simulink model "JoshTestingOCTModel"  (R2018b)
settings: Solver=VariableStepAuto  StartTime=0.0  StopTime=simParams.duration.Value  FixedStep=0.01  MaxStep=0.1*sqrt(simParams.lengthScaleFactor.Value)  RelTol=1e-3  AbsTol=1e-3
undefined symbols (not defined in the file): dragTurbine, dragTurbine_ul, env, flightController, FLIGHTCONTROLLER, flightController_cl, fltCtrl, fluidDynamicSurface, fluidDynamicSurface_cl, fuselage, fuselage_cl, initializeBussesFromBlock, initializeVariantsFromBlock, pathFollowingController, pathFollowingController_cl, plant, plant_cl, sixDoFDynamics, sixDoFDynamics_cl, sixDoFDynamicsCoupled, surfaceCoefficients, surfaceCoefficients_ul, tethersMoment, tethersMoment_cl, thrAttachPtKinematics, thrAttachPtKinematics_ul, vehicle, vehicle_cl, vehicleLE, vehicleLE_cl, vhcl
libraries: vrlib x18, dspstat3 x3, vectorNormalizer_ul x3, localApparentWind_ul x3, xProdMatrix_ul x2, dynamicPressure_ul x2, dsppolyfun x2, animation_cl x1, environment_cl x1, oneTetherThreeSurfaceCtrl_cl x1, courseFollow_cl x1, ctrlAllocMatrixLE_cl x1
(part 1 of 2)
PreSaveFcn:
  | % Callback to reset the view so that the
  | % the next person to open isn't totally lost.
  | hilite_system('OCTModel/plant');
  | hilite_system('OCTModel/plant','none');
  | set_param(gcs,'Zoomfactor','fit to view')
settings Model: SimulationMode=accelerator  ExtModeTrigDuration=100  Creator=mcobb  LastModifiedBy=jldanie5
settings SolverCC: AlgebraicLoopSolver=LineSearch  SolverResetMethod=Robust
settings DataIOCC: SaveOutput=off  DSMLogging=off  StateSaveName=tmp_raccel_xout
settings OptimizationCC: EfficientMapNaN2IntZero=off
settings DebuggingCC: SignalRangeChecking=error  AlgebraicLoopMsg=none  ArtificialAlgebraicLoopMsg=none
settings HardwareCC: TargetBitPerPointer=64  TargetBitPerSizeT=64  TargetBitPerPtrDiffT=64  TargetLongLongMode=on  TargetIntDivRoundTo=Zero  TargetEndianess=LittleEndian  TargetWordSize=64  TargetHWDeviceType=MATLAB Host  ProdEqTarget=off
settings CodeAppCC: MaxIdLength=128
settings GRTTargetCC: TargetLangStandard=C89/C90 (ANSI)  CombineOutputUpdateFcns=off  GRTInterface=on

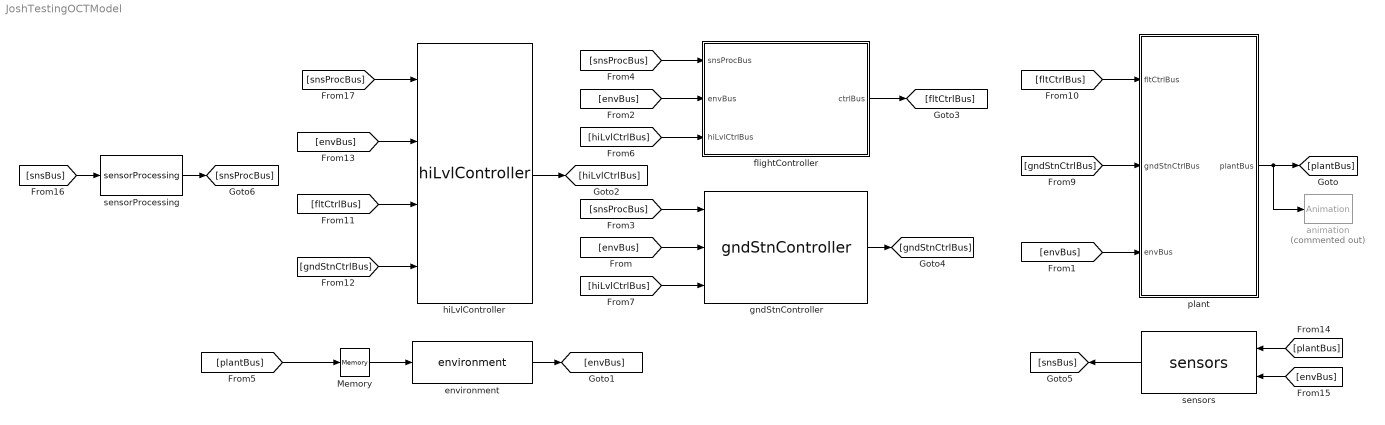
== system JoshTestingOCTModel ==
  Memory : Memory
  animation : animation_cl/Animation  Commented=on  animSampleTime=0.1  scaleFactor=scaleFactor  elevation=45  radius=500  vidLogEnbl=off  vidDims=[240 480]*2
  environment : environment_cl/environment  SystemSampleTime=-1
  flightController : Subsystem  AncestorBlock=flightController_cl/flightController  LoadFcn=initializeVariantsFromBlock(gcb)  InitFcn=initializeVariantsFromBlock(gcb)  StartFcn=initializeVariantsFromBlock(gcb)  Variant=on
      settings: PreSaveFcn=initializeVariantsFromBlock(gcb)
  gndStnController : gndStnController_cl/gndStnController  SystemSampleTime=-1
      link override anchorTetherCtrl: ctrl=gndCtrl
  hiLvlController : hiLvlController_cl/hiLvlController  SystemSampleTime=-1
  plant : Subsystem  AncestorBlock=plant_cl/plant  LoadFcn=initializeBussesFromBlock(gcb)  InitFcn=initializeBussesFromBlock(gcb)  StartFcn=initializeBussesFromBlock(gcb)  VariantControl=VSS_plant_modularPlant
  sensorProcessing : sensorProcessing_cl/sensorProcessing  SystemSampleTime=-1
  sensors : sensors_cl/sensors  SystemSampleTime=-1
  wires:
  environment/1 -> [envBus]
  [envBus] -> gndStnController/2
  [envBus] -> plant/3(envBus)
  [snsProcBus] -> gndStnController/1
  [snsProcBus] -> flightController/1(snsProcBus)
  [snsProcBus] -> hiLvlController/1
  flightController/1(ctrlBus) -> [fltCtrlBus]
  gndStnController/1 -> [gndStnCtrlBus]
  [gndStnCtrlBus] -> plant/2(gndStnCtrlBus)
  [fltCtrlBus] -> plant/1(fltCtrlBus)
  [envBus] -> hiLvlController/2
  [fltCtrlBus] -> hiLvlController/3
  [gndStnCtrlBus] -> hiLvlController/4
  [plantBus] -> Memory/1
  [hiLvlCtrlBus] -> flightController/3(hiLvlCtrlBus)
  [hiLvlCtrlBus] -> gndStnController/3
  plant/1(plantBus) -> [plantBus], animation/1
  hiLvlController/1 -> [hiLvlCtrlBus]
  Memory/1 -> environment/1
  [envBus] -> flightController/2(envBus)
  [plantBus] -> sensors/1
  [envBus] -> sensors/2
  sensors/1 -> [snsBus]
  [snsBus] -> sensorProcessing/1
  sensorProcessing/1 -> [snsProcBus]

== system JoshTestingOCTModel/flightController ==
  snsProcBus : Inport  OutDataTypeStr=Bus: sensorsProcessingBus
  envBus : Inport  Port=2  OutDataTypeStr=Bus: envBus
  hiLvlCtrlBus : Inport  Port=3  OutDataTypeStr=Bus: hiLvlCtrlBus
  oneTetherThreeSurfaceCtrl : oneTetherThreeSurfaceCtrl_cl/oneTetherThreeSurfaceCtrl  SystemSampleTime=-1  VariantControl=strcmpi(FLIGHTCONTROLLER,'oneTetherThreeSurfaceCtrl')
  pathFollowingController : Subsystem  AncestorBlock=pathFollowingController_cl/pathFollowingController  LoadFcn=initializeBussesFromBlock(gcb)  InitFcn=initializeBussesFromBlock(gcb)  StartFcn=initializeBussesFromBlock(gcb)  VariantControl=strcmpi(FLIGHTCONTROLLER,'pathFollowingController')  mask{initPosForInitSStar=vhcl.initPosVecGnd.Value, fluidDensity=env.water.density.Value, pathCtrl=fltCtrl, aeroStruct=vhcl.struct('OCT.aeroSurfLE')}
      mask prompts: initPosForInitSStar "Initial Position"; fluidDensity "Fluid Density"; pathCtrl "Controller"; aeroStruct "Aerodynamic Structure"
      settings: MinAlgLoopOccurrences=on
      mask DialogControl Container3 Prompt: courseFollow Params
      mask DialogControl Container4 Prompt: setpointToOutput Params
  takeoffToLanding : takeoffToLanding_cl/takeoffToLanding  VariantControl=strcmpi(FLIGHTCONTROLLER,'takeoffToLanding')  initPosForInitSStar=vhcl.initPosVecGnd.Value  fluidDensity=env.water.density.Value  pathCtrl=fltCtrl  aeroStruct=vhcl.struct('OCT.aeroSurf')
  threeTetherThreeSurfaceCtrl : threeTetherThreeSurfaceCtrl_cl/threeTetherThreeSurfaceCtrl  VariantControl=strcmpi(FLIGHTCONTROLLER,'threeTetherThreeSurfaceCtrl')  ctrl=fltCtrl
  ctrlBus : Outport  OutDataTypeStr=Bus: fltCtrlBus

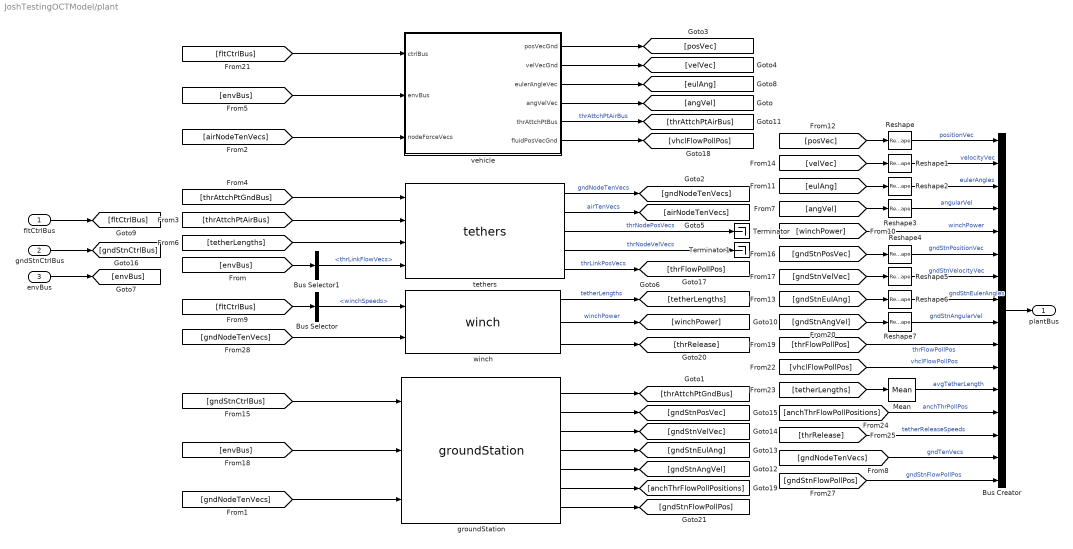
== system JoshTestingOCTModel/plant ==
  fltCtrlBus : Inport  OutDataTypeStr=Bus: fltCtrlBus
  gndStnCtrlBus : Inport  Port=2  OutDataTypeStr=Bus: gndStnCtrlBus
  envBus : Inport  Port=3  OutDataTypeStr=Bus: envBus
  Bus Creator : BusCreator  Inputs=16  OutDataTypeStr=Bus: plantBus  NonVirtualBus=on
  Bus Selector : BusSelector  OutputSignals=winchSpeeds
  Bus Selector1 : BusSelector  OutputSignals=thrLinkFlowVecs
  Mean : dspstat3/Mean  run=off  InputProcessing=Columns as channels (frame based)  reset_popup=None  directionMode=Each column  dimension=1  roiEnable=off  roiType=Rectangles  roiPortion=Entire ROI  roiOutput=Individual statistics for each ROI  roiFlag=off  roundingMode=Floor  overflowMode=off  outputDataTypeStr=Inherit: Same as accumulator  outputMin=[]  outputMax=[]  outputLastDataTypeStr=Inherit: Same as accumulator
  Reshape{,1..7} (8 alike) : Reshape  OutputDimensionality=Column vector (2-D)
  Terminator : Terminator
  Terminator1 : Terminator
  groundStation : groundStation_cl/groundStation  numNodes=2
  tethers : tethers_cl/tethers  SystemSampleTime=-1
  vehicle : Subsystem  AncestorBlock=vehicle_cl/vehicle  LoadFcn=initializeVariantsFromBlock(gcb)  InitFcn=initializeVariantsFromBlock(gcb)  StartFcn=initializeVariantsFromBlock(gcb)  Variant=on
      settings: PreSaveFcn=initializeVariantsFromBlock(gcb)
  winch : winch_cl/winch  SystemSampleTime=-1
  plantBus : Outport  OutDataTypeStr=Bus: plantBus
  wires:
  [gndNodeTenVecs] -> winch/2
  tethers/5 -> [thrFlowPollPos]  "thrLinkPosVecs"
  [gndStnFlowPollPos] -> Bus Creator/16  "gndStnFlowPollPos"
  groundStation/7 -> [gndStnFlowPollPos]
  [gndNodeTenVecs] -> Bus Creator/15  "gndTenVecs"
  [thrRelease] -> Bus Creator/14  "tetherReleaseSpeeds"
  [anchThrFlowPollPositions] -> Bus Creator/13  "anchThrPollPos"
  groundStation/6 -> [anchThrFlowPollPositions]
  Mean/1 -> Bus Creator/12  "avgTetherLength"
  [tetherLengths] -> Mean/1
  Bus Selector1/1 -> tethers/4  "<thrLinkFlowVecs>"
  [vhclFlowPollPos] -> Bus Creator/11  "vhclFlowPollPos"
  vehicle/6(fluidPosVecGnd) -> [vhclFlowPollPos]
  [thrFlowPollPos] -> Bus Creator/10  "thrFlowPollPos"
  tethers/4 -> Terminator1/1  "thrNodeVelVecs"
  winch/3 -> [thrRelease]
  Bus Selector/1 -> winch/1  "<winchSpeeds>"
  gndStnCtrlBus/1 -> [gndStnCtrlBus]
  groundStation/5 -> [gndStnAngVel]
  groundStation/4 -> [gndStnEulAng]
  groundStation/3 -> [gndStnVelVec]
  groundStation/2 -> [gndStnPosVec]
  Reshape7/1 -> Bus Creator/9  "gndStnAngularVel"
  Reshape6/1 -> Bus Creator/8  "gndStnEulerAngles"
  Reshape5/1 -> Bus Creator/7  "gndStnVelocityVec"
  Reshape4/1 -> Bus Creator/6  "gndStnPositionVec"
  [gndStnPosVec] -> Reshape4/1
  [gndStnVelVec] -> Reshape5/1
  [gndStnEulAng] -> Reshape6/1
  [gndStnAngVel] -> Reshape7/1
  [winchPower] -> Bus Creator/5  "winchPower"
  winch/2 -> [winchPower]  "winchPower"
  Reshape3/1 -> Bus Creator/4  "angularVel"
  [angVel] -> Reshape3/1
  [fltCtrlBus] -> Bus Selector/1
  [envBus] -> vehicle/2(envBus)
  [fltCtrlBus] -> vehicle/1(ctrlBus)
  [gndStnCtrlBus] -> groundStation/1
  [envBus] -> groundStation/2
  [tetherLengths] -> tethers/3
  [thrAttchPtGndBus] -> tethers/1
  [thrAttchPtAirBus] -> tethers/2
  [airNodeTenVecs] -> vehicle/3(nodeForceVecs)
  [gndNodeTenVecs] -> groundStation/3
  tethers/3 -> Terminator/1  "thrNodePosVecs"
  tethers/2 -> [airNodeTenVecs]  "airTenVecs"
  tethers/1 -> [gndNodeTenVecs]  "gndNodeTenVecs"
  groundStation/1 -> [thrAttchPtGndBus]
  [envBus] -> Bus Selector1/1
  vehicle/4(angVelVec) -> [angVel]
  vehicle/2(velVecGnd) -> [velVec]
  vehicle/5(thrAttchPtBus) -> [thrAttchPtAirBus]  "thrAttchPtAirBus"
  vehicle/1(posVecGnd) -> [posVec]
  vehicle/3(eulerAngleVec) -> [eulAng]
  [eulAng] -> Reshape2/1
  [velVec] -> Reshape1/1
  [posVec] -> Reshape/1
  winch/1 -> [tetherLengths]  "tetherLengths"
  Reshape1/1 -> Bus Creator/2  "velocityVec"
  Reshape2/1 -> Bus Creator/3  "eulerAngles"
  Reshape/1 -> Bus Creator/1  "positionVec"
  Bus Creator/1 -> plantBus/1
  fltCtrlBus/1 -> [fltCtrlBus]
  envBus/1 -> [envBus]

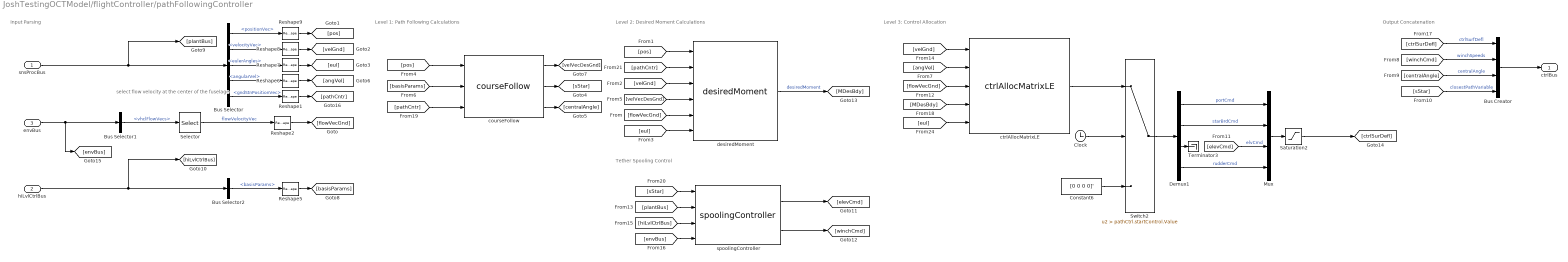
== system JoshTestingOCTModel/flightController/pathFollowingController ==
  note: Input Parsing
  note: Level 1: Path Following Calculations
  note: Level 2: Desired Moment Calculations
  note: Tether Spooling Control
  note: Output Concatenation
  note: Level 3: Control Allocation
  note: select flow velocity at the center of the fuselage
  snsProcBus : Inport  OutDataTypeStr=Bus: sensorsProcessingBus
  hiLvlCtrlBus : Inport  Port=2  OutDataTypeStr=Bus: hiLvlCtrlBus
  envBus : Inport  Port=3  OutDataTypeStr=Bus: envBus
  Bus Creator : BusCreator  Inputs=4  OutDataTypeStr=Bus: fltCtrlBus
      settings: InheritFromInputs=off
  Bus Selector : BusSelector  OutputSignals=positionVec,velocityVec,eulerAngles,angularVel,gndStnPositionVec
  Bus Selector1 : BusSelector  OutputSignals=vhclFlowVecs
  Bus Selector2 : BusSelector  OutputSignals=basisParams
  Clock : Clock
  Constant6 : Constant  Value=[0 0 0 0]'
  Demux1 : Demux
  Mux : Mux
  Reshape{1..2,5..9} (7 alike) : Reshape  OutputDimensionality=Column vector (2-D)
  Saturation2 : Saturate  UpperLimit=pathCtrl.controlSigMax.upperLimit.Value  LowerLimit=pathCtrl.controlSigMax.lowerLimit.Value
  Selector : Selector  NumberOfDimensions=2  InputPortWidth=3  IndexOptions=Select all,Index vector (dialog)  Indices=[1 3],5  OutputSizes=1,1
  Switch2 : Switch  Criteria=u2 > Threshold  Threshold=pathCtrl.startControl.Value
  Terminator3 : Terminator
  courseFollow : courseFollow_cl/courseFollow  SystemSampleTime=-1
  ctrlAllocMatrixLE : ctrlAllocMatrixLE_cl/ctrlAllocMatrixLE  aeroStruct=aeroStruct  fluidDensity=fluidDensity  ctrlUpMax=pathCtrl.controlSigMax.upperLimit.Value  ctrlDnMax=pathCtrl.controlSigMax.lowerLimit.Value
  desiredMoment : setpointToOutput_cl/desiredMoment  SystemSampleTime=-1
  spoolingController : spoolingController_cl/spoolingController  SystemSampleTime=-1
  ctrlBus : Outport  OutDataTypeStr=Bus: fltCtrlBus
  wires:
  [basisParams] -> courseFollow/2
  [flowVecGnd] -> desiredMoment/5
  [eul] -> desiredMoment/6
  [velVecDesGnd] -> desiredMoment/4
  [velGnd] -> desiredMoment/3
  [pathCntr] -> desiredMoment/2
  [pos] -> desiredMoment/1
  [pathCntr] -> courseFollow/3
  Bus Selector/5 -> Reshape1/1  "<gndStnPositionVec>"
  Reshape1/1 -> [pathCntr]
  [envBus] -> spoolingController/4
  spoolingController/2 -> [winchCmd]
  spoolingController/1 -> [elevCmd]
  Bus Selector1/1 -> Selector/1  "<vhclFlowVecs>"
  [hiLvlCtrlBus] -> spoolingController/3
  [plantBus] -> spoolingController/2
  [sStar] -> spoolingController/1
  envBus/1 -> Bus Selector1/1, [envBus]
  Selector/1 -> Reshape2/1  "flowVelocityVec"
  [eul] -> ctrlAllocMatrixLE/5
  Reshape9/1 -> [pos]
  Reshape8/1 -> [velGnd]
  Reshape7/1 -> [eul]
  Reshape6/1 -> [angVel]
  Reshape2/1 -> [flowVecGnd]
  Saturation2/1 -> [ctrlSurDefl]
  Reshape5/1 -> [basisParams]
  Bus Selector2/1 -> Reshape5/1  "<basisParams>"
  [ctrlSurDefl] -> Bus Creator/1  "ctrlSurfDefl"
  ctrlAllocMatrixLE/1 -> Switch2/1
  [MDesBdy] -> ctrlAllocMatrixLE/4
  Constant6/1 -> Switch2/3
  Switch2/1 -> Demux1/1
  Clock/1 -> Switch2/2
  Demux1/2 -> Mux/2  "starBrdCmd"
  Demux1/1 -> Mux/1  "portCmd"
  Demux1/4 -> Mux/4  "rudderCmd"
  Demux1/3 -> Terminator3/1
  Mux/1 -> Saturation2/1
  [elevCmd] -> Mux/3  "elvCmd"
  [flowVecGnd] -> ctrlAllocMatrixLE/3
  [velGnd] -> ctrlAllocMatrixLE/1
  [angVel] -> ctrlAllocMatrixLE/2
  Bus Selector/4 -> Reshape6/1  "<angularVel>"
  desiredMoment/1 -> [MDesBdy]  "desiredMoment"
  courseFollow/3 -> [centralAngle]
  [sStar] -> Bus Creator/4  "closestPathVariable"
  [centralAngle] -> Bus Creator/3  "centralAngle"
  hiLvlCtrlBus/1 -> Bus Selector2/1, [hiLvlCtrlBus]
  courseFollow/2 -> [sStar]
  [winchCmd] -> Bus Creator/2  "winchSpeeds"
  Bus Creator/1 -> ctrlBus/1
  [pos] -> courseFollow/1
  Bus Selector/3 -> Reshape7/1  "<eulerAngles>"
  Bus Selector/1 -> Reshape9/1  "<positionVec>"
  Bus Selector/2 -> Reshape8/1  "<velocityVec>"
  snsProcBus/1 -> Bus Selector/1, [plantBus]
  courseFollow/1 -> [velVecDesGnd]

== system JoshTestingOCTModel/plant/vehicle ==
  ctrlBus : Inport  OutDataTypeStr=Bus: fltCtrlBus
  envBus : Inport  Port=2  OutDataTypeStr=Bus: envBus
  nodeForceVecs : Inport  Port=3
  vehicle000 : vehicle000_cl/vehicle000  VariantControl=VSS_vehicle_vehicle000  vcl=vhcl  rho=env.water.density.Value  grav=env.gravAccel.Value
  vehicleLETest : Subsystem  AncestorBlock=vehicleLE_cl/vehicleLE  VariantControl=VSS_vehicle_vehicleLETest  mask{vcl=vhcl, rho=env.water.density.Value, grav=env.gravAccel.Value}
      mask prompts: vcl "Vehicle"; rho "Density"; grav "Gravity"
      mask DialogControl Container9 Prompt: General
      mask DialogControl Container5 Prompt: Vehicle object (OCT.vehicle)
      mask DialogControl ParameterGroupVar Prompt: Environment Object (OCT.env)
      mask Display:
      | image('kite.jpg',[100 100 601 528]/4,'on')
      | 
      | port_label('input',1,'ctrlBus')
      | port_label('input',2,'envBus')
      | port_label('input',3,'nodeForceVecs')
      | 
      | port_label('output',1,'posVecGnd')
      | port_label('output',2,'velVecGnd')
      | port_label('output',3,'eulAng')
      | port_label('output',4,'angVelVec')
      | port_label('output',5,'thrAttchPtBus')
      | port_label('output',6,'fluidPosVecGnd')
  posVecGnd : Outport
  velVecGnd : Outport  Port=2
  eulerAngleVec : Outport  Port=3
  angVelVec : Outport  Port=4
  thrAttchPtBus : Outport  Port=5
  fluidPosVecGnd : Outport  Port=6

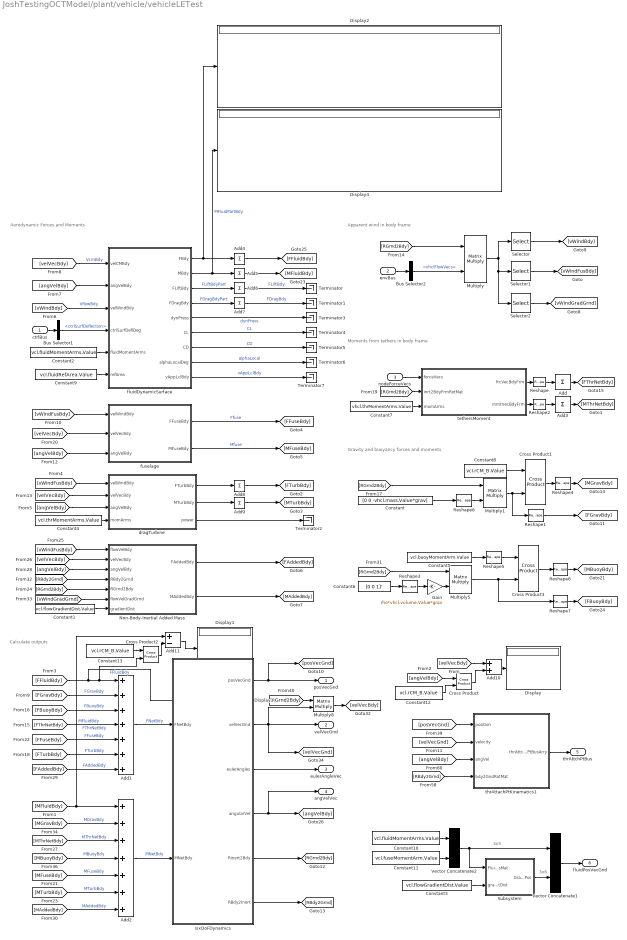
== system JoshTestingOCTModel/plant/vehicle/vehicleLETest ==
  note: Aerodynamic Forces and Moments
  note: Moments from tethers in body frame
  note: Gravity and buoyancy forces and moments
  note: Apparent wind in body frame
  note: Calculate outputs
  note: 3x5
  note: 3x6
  ctrlBus : Inport  OutDataTypeStr=Bus: fltCtrlBus
  envBus : Inport  Port=2  OutDataTypeStr=Bus: envBus
  nodeForceVecs : Inport  Port=3
  Add : Sum  Inputs=+  CollapseMode=Specified dimension  CollapseDim=2
  Add1 : Sum  Inputs=+++++++
  Add10 : Sum
  Add11 : Sum  Inputs=+-
  Add2 : Sum  Inputs=+++++++
  Add3 : Sum  Inputs=+  CollapseMode=Specified dimension  CollapseDim=2
  Add{4..9} (6 alike) : Sum  Inputs=1  CollapseMode=Specified dimension  CollapseDim=2
  Bus Selector1 : BusSelector  OutputSignals=ctrlSurfDeflection
  Bus Selector2 : BusSelector  OutputSignals=vhclFlowVecs
  Constant : Constant  Value=[0 0 -vhcl.mass.Value*grav]
  Constant1 : Constant  Value=vcl.flowGradientDist.Value
  Constant10 : Constant  Value=vcl.fluidMomentArms.Value
  Constant11 : Constant  Value=vcl.fuseMomentArm.Value
  Constant12 : Constant  Value=vcl.rCM_B.Value
  Constant13 : Constant  Value=vcl.rCM_B.Value
  Constant2 : Constant  Value=vcl.fluidMomentArms.Value
  Constant3 : Constant  Value=vcl.flowGradientDist.Value
  Constant4 : Constant  Value=vcl.thrMomentArms.Value  VectorParams1D=off
  Constant5 : Constant  Value=vcl.buoyMomentArm.Value
  Constant6 : Constant  Value=[0 0 1]'
  Constant7 : Constant  Value=vhcl.thrMomentArms.Value
  Constant8 : Constant  Value=vcl.rCM_B.Value
  Constant9 : Constant  Value=vcl.fluidRefArea.Value
  Cross Product{,1..3} (4 alike) : vrlib/Utilities/Cross Product
      settings: SourceProductBaseCode=VR
  Display{,1..4} (5 alike) : Display
  Gain : Gain  Gain=rho*vhcl.volume.Value*grav
  Multiply{,1,5,8} (4 alike) : Product  Multiplication=Matrix(*)
  Non-Body-Inertial Added Mass : Subsystem  AncestorBlock=addedMass_cl/Non-Body-Inertial Added Mass  mask{MaMat=vcl.Ma6x6_B.Value}
      mask prompts: MaMat "Added Mass Matrix"
  Reshape : Reshape  OutputDimensionality=Customize  OutputDimensions=[3 vcl.numTethers.Value]
  Reshape{1,3..8} (7 alike) : Reshape  OutputDimensionality=Column vector (2-D)
  Reshape2 : Reshape  OutputDimensionality=Customize  OutputDimensions=[3 vcl.numTethers.Value]
  Selector : Selector  NumberOfDimensions=2  InputPortWidth=3  IndexOptions=Select all,Index vector (dialog)  Indices=[1 3],1:4  OutputSizes=1,1
  Selector1 : Selector  NumberOfDimensions=2  InputPortWidth=3  IndexOptions=Select all,Index vector (dialog)  Indices=[1 3],5  OutputSizes=1,1
  Selector2 : Selector  NumberOfDimensions=2  InputPortWidth=3  IndexOptions=Select all,Index vector (dialog)  Indices=[1 3],6:11  OutputSizes=1,1
  Subsystem : Subsystem
  Terminator{,1..7} (8 alike) : Terminator
  Vector Concatenate1 : Concatenate  Mode=Multidimensional array  ConcatenateDimension=2
  Vector Concatenate2 : Concatenate  Mode=Multidimensional array  ConcatenateDimension=2
  dragTurbine : Subsystem  AncestorBlock=dragTurbine_ul/dragTurbine  TreatAsAtomicUnit=on  mask{rho_fluid=rho, turb_struct=vcl.struct('OCT.turb'), momArms=0}
      mask prompts: rho_fluid "Fluid density"; turb_struct "Turbines structure"; momArms "Turbine Moment Arms"
  fluidDynamicSurface : Subsystem  AncestorBlock=fluidDynamicSurface_cl/fluidDynamicSurface  mask{aeroStruct=vcl.struct('OCT.aeroSurfLE'), fluidDensity=env.water.density.Value}
      mask prompts: aeroStruct "Aerodynamic surface structure"; fluidDensity "Fluid density"
      mask help:
      | Input must be an 1×N struct array with fields:
      |     refArea
      |     aeroCentPosVec
      |     spanUnitVec
      |     chordUnitVec
      |     CL
      |     CD
      |     alpha
      |     GainCL
      |     GainCD
      |
      | where N is the number of aerodynamic surfaces
      settings: MinAlgLoopOccurrences=on
  fuselage : Subsystem  AncestorBlock=fuselage_cl/fuselage  mask{momArm=vcl.fuseMomentArm.Value, fus=vcl.fuse, fusRhoDa=rho}
      mask prompts: momArm "Fuselage Moment Arm"; fus "Fuselage"; fusRhoDa "Density"
      mask DialogControl Container4 Prompt: General
      mask DialogControl Container9 Prompt: Fuselage object (OCT.fuselage)
      mask DialogControl Container8 Prompt: Environment Object (OCT.env)
  sixDoFDynamics : Subsystem  AncestorBlock=sixDoFDynamics_cl/sixDoFDynamics  LoadFcn=initializeVariantsFromBlock(gcb)  InitFcn=initializeVariantsFromBlock(gcb)  Variant=on  mask{vcl=vcl}
      mask prompts: vcl "vehicle object"
  tethersMoment : Subsystem  AncestorBlock=tethersMoment_cl/tethersMoment  mask{arms=vcl.struct('OCT.thrAttchLE')}
      mask prompts: arms "Moment arm(s)"
  thrAttachPtKinematics1 : Subsystem  AncestorBlock=thrAttachPtKinematics_ul/thrAttachPtKinematics  InitFcn=thrAttachPtKinematics_init  mask{atchPts=vcl.struct('OCT.thrAttchLE')}
      mask prompts: atchPts "Tether attachment point vec in platform frame"
      mask init:
      | thrAttachPtKinematics_init
  posVecGnd : Outport
  velVecGnd : Outport  Port=2
  eulerAngleVec : Outport  Port=3
  angVelVec : Outport  Port=4
  thrAttchPtBus : Outport  Port=5
  fluidPosVecGnd : Outport  Port=6
  wires:
  Add10/1 -> Display/1
  Cross Product/1 -> Add10/2
  [velVecBdy] -> Add10/1
  Constant12/1 -> Cross Product/2
  [angVelBdy] -> Cross Product/1
  Non-Body-Inertial Added Mass/2(MAddedBdy) -> [MAddedBdy]
  sixDoFDynamics/4(angularVel) -> angVelVec/1, [angVelBdy]
  Vector Concatenate1/1 -> fluidPosVecGnd/1
  Subsystem/1(GradientFlowPos) -> Vector Concatenate1/2
  Constant3/1 -> Subsystem/2(gradientDist)
  Vector Concatenate2/1 -> Vector Concatenate1/1, Subsystem/1(FluidCentPosMat)
  Constant11/1 -> Vector Concatenate2/2
  Constant10/1 -> Vector Concatenate2/1
  [RBdy2Grnd] -> thrAttachPtKinematics1/4(bdy2GndRotMat)
  [angVelBdy] -> thrAttachPtKinematics1/3(angVel)
  [velVecGnd] -> thrAttachPtKinematics1/2(velocity)
  [posVecGnd] -> thrAttachPtKinematics1/1(position)
  sixDoFDynamics/6(RBdy2Inert) -> [RBdy2Grnd]
  sixDoFDynamics/5(Rinert2Bdy) -> [RGrnd2Bdy]
  Add2/1 -> sixDoFDynamics/2(MNetBdy)  "MNetBdy"
  [MAddedBdy] -> Add2/7  "MAddedBdy"
  [MTurbBdy] -> Add2/6  "MTurbBdy"
  [MFuseBdy] -> Add2/5  "MFuseBdy"
  [MBuoyBdy] -> Add2/4  "MBuoyBdy"
  [MThrNetBdy] -> Add2/3  "MThrNetBdy"
  [MGravBdy] -> Add2/2  "MGravBdy"
  [MFluidBdy] -> Add11/1, Add2/1  "MFluidBdy"
  Add1/1 -> sixDoFDynamics/1(FNetBdy)  "FNetBdy"
  [FAddedBdy] -> Add1/7  "FAddedBdy"
  [FTurbBdy] -> Add1/6  "FTurbBdy"
  [FFuseBdy] -> Add1/5  "FFuseBdy"
  [FThrNetBdy] -> Add1/4  "FThrNetBdy"
  [FBuoyBdy] -> Add1/3  "FBuoyBdy"
  [FGravBdy] -> Add1/2  "FGravBdy"
  [FFluidBdy] -> Display3/1, Cross Product2/2, Add1/1  "FFluidBdy"
  Multiply8/1 -> [velVecBdy]
  [RGrnd2Bdy] -> Multiply8/1
  Selector2/1 -> [vWindGradGrnd]
  Selector1/1 -> [vWindFusBdy]
  Selector/1 -> [vWindBdy]
  Multiply/1 -> Selector1/1, Selector2/1, Selector/1
  Bus Selector2/1 -> Multiply/2  "<vhclFlowVecs>"
  envBus/1 -> Bus Selector2/1
  [RGrnd2Bdy] -> Multiply/1
  Add3/1 -> [MThrNetBdy]
  Add/1 -> [FThrNetBdy]
  Reshape2/1 -> Add3/1
  Reshape/1 -> Add/1
  tethersMoment/2(mmtVecBdyFrm) -> Reshape2/1
  tethersMoment/1(frcVecBdyFrm) -> Reshape/1
  nodeForceVecs/1 -> tethersMoment/1(forceVecs)
  [RGrnd2Bdy] -> tethersMoment/2(inrt2BdyFrmRotMat)
  Constant7/1 -> tethersMoment/3(momArms)
  Reshape4/1 -> [MGravBdy]
  Cross Product1/1 -> Reshape4/1
  Constant8/1 -> Cross Product1/1
  Reshape8/1 -> Multiply1/2
  [RGrnd2Bdy] -> Multiply1/1
  Constant/1 -> Reshape8/1
  fuselage/2(MFuseBdy) -> [MFuseBdy]  "Mfuse"
  fuselage/1(FFuseBdy) -> [FFuseBdy]  "Ffuse"
  Multiply1/1 -> Cross Product1/2, Reshape1/1
  Reshape1/1 -> [FGravBdy]
  Reshape7/1 -> [FBuoyBdy]
  Multiply5/1 -> Cross Product3/2, Reshape7/1
  Reshape6/1 -> [MBuoyBdy]
  Cross Product3/1 -> Reshape6/1
  Reshape5/1 -> Cross Product3/1
  Constant5/1 -> Reshape5/1
  Gain/1 -> Multiply5/2
  [RGrnd2Bdy] -> Multiply5/1
  Reshape3/1 -> Gain/1
  Constant6/1 -> Reshape3/1
  Non-Body-Inertial Added Mass/1(FAddedBdy) -> [FAddedBdy]
  Constant1/1 -> Non-Body-Inertial Added Mass/7(gradientDist)
  [vWindGradGrnd] -> Non-Body-Inertial Added Mass/6(flowVelGradGrnd)
  [RGrnd2Bdy] -> Non-Body-Inertial Added Mass/5(RGrnd2Bdy)
  [RBdy2Grnd] -> Non-Body-Inertial Added Mass/4(RBdy2Grnd)
  [angVelBdy] -> Non-Body-Inertial Added Mass/3(angVelBdy)
  [velVecBdy] -> Non-Body-Inertial Added Mass/2(velVecBdy)
  [vWindFusBdy] -> Non-Body-Inertial Added Mass/1("flowVelBdy ")
  dragTurbine/3(power) -> Terminator2/1
  Add9/1 -> [MTurbBdy]
  Add8/1 -> [FTurbBdy]
  dragTurbine/2(MTurbBdy) -> Add9/1
  dragTurbine/1(FTurbBdy) -> Add8/1
  Constant4/1 -> dragTurbine/4(momArms)
  [angVelBdy] -> dragTurbine/3(angVelBdy)
  [velVecBdy] -> dragTurbine/2(velVecBdy)
  [vWindFusBdy] -> dragTurbine/1(velWindBdy)
  [angVelBdy] -> fuselage/3(angVelBdy)
  [velVecBdy] -> fuselage/2(velVecBdy)
  [vWindFusBdy] -> fuselage/1(velWindBdy)
  Constant9/1 -> fluidDynamicSurface/6(refArea)
  ctrlBus/1 -> Bus Selector1/1
  Bus Selector1/1 -> fluidDynamicSurface/4(ctrlSurfDeflDeg)  "<ctrlSurfDeflection>"
  [vWindBdy] -> fluidDynamicSurface/3(velWindBdy)  "VflowBdy"
  [angVelBdy] -> fluidDynamicSurface/2(angVelBdy)
  [velVecBdy] -> fluidDynamicSurface/1(velCMBdy)  "VcmBdy"
  Add7/1 -> Terminator1/1  "FDragBdy"
  Add6/1 -> Terminator/1  "FLiftBdy"
  Add5/1 -> [MFluidBdy]
  Add4/1 -> [FFluidBdy]
  fluidDynamicSurface/9(vAppLclBdy) -> Terminator7/1  "vAppLclBdy"
  fluidDynamicSurface/8(alphaLocalDeg) -> Terminator6/1  "alphaLocal"
  fluidDynamicSurface/7(CD) -> Terminator5/1  "CD"
  fluidDynamicSurface/6(CL) -> Terminator4/1  "CL"
  fluidDynamicSurface/5(dynPress) -> Terminator3/1  "dynPress"
  fluidDynamicSurface/4(FDragBdy) -> Add7/1  "FDragBdyPart"
  fluidDynamicSurface/3(FLiftBdy) -> Add6/1  "FLiftBdyPart"
  fluidDynamicSurface/2(MBdy) -> Display4/1, Add5/1  "MFluidPartBdy"
  Constant2/1 -> fluidDynamicSurface/5(fluidMomentArms)
  fluidDynamicSurface/1(FBdy) -> Display2/1, Add4/1
  thrAttachPtKinematics1/1(thrAttchPtBusArry) -> thrAttchPtBus/1
  sixDoFDynamics/2(velVecGnd) -> velVecGnd/1, [velVecGnd], Multiply8/2
  sixDoFDynamics/1(posVecGnd) -> posVecGnd/1, [posVecGnd]
  sixDoFDynamics/3(eulerAngles) -> eulerAngleVec/1
  Cross Product2/1 -> Add11/2
  Add11/1 -> Display1/1
  Constant13/1 -> Cross Product2/1

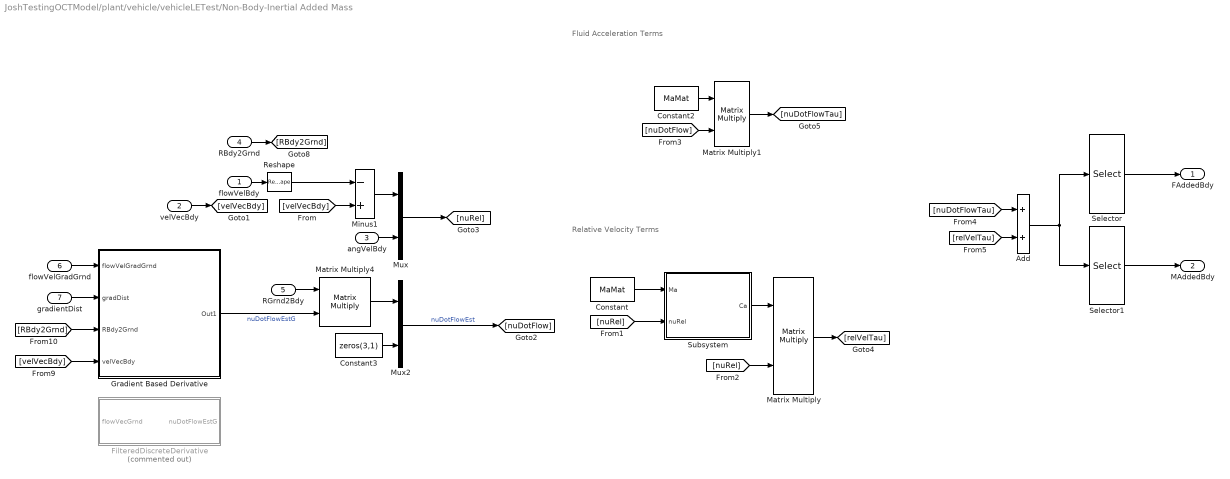
== system JoshTestingOCTModel/plant/vehicle/vehicleLETest/Non-Body-Inertial Added Mass ==
  note: Fluid Acceleration Terms
  note: Relative Velocity Terms
  "flowVelBdy " : Inport
  velVecBdy : Inport  Port=2
  angVelBdy : Inport  Port=3
  RBdy2Grnd : Inport  Port=4
  RGrnd2Bdy : Inport  Port=5
  flowVelGradGrnd : Inport  Port=6
  gradientDist : Inport  Port=7
  Add : Sum
  Constant : Constant  Value=MaMat
  Constant2 : Constant  Value=MaMat
  Constant3 : Constant  Value=zeros(3,1)
  FilteredDiscreteDerivative : Subsystem  Commented=on
  Gradient Based Derivative : Subsystem
  Matrix Multiply : Product  Multiplication=Matrix(*)
  Matrix Multiply1 : Product  Multiplication=Matrix(*)
  Matrix Multiply4 : Product  Multiplication=Matrix(*)
  Minus1 : Sum  Inputs=-+
  Mux : Mux  Inputs=2
  Mux2 : Mux  Inputs=2
  Reshape : Reshape  OutputDimensionality=Column vector (2-D)
  Selector : Selector  InputPortWidth=6  IndexOptions=Index vector (dialog)  Indices=[1 2 3]  OutputSizes=1
  Selector1 : Selector  InputPortWidth=6  IndexOptions=Index vector (dialog)  Indices=[4 5 6]  OutputSizes=1
  Subsystem : Subsystem
  FAddedBdy : Outport
  MAddedBdy : Outport  Port=2
  wires:
  Reshape/1 -> Minus1/1
  Gradient Based Derivative/1(Out1) -> Matrix Multiply4/2  "nuDotFlowEstG"
  RBdy2Grnd/1 -> [RBdy2Grnd]
  [velVecBdy] -> Gradient Based Derivative/4(velVecBdy)
  [RBdy2Grnd] -> Gradient Based Derivative/3(RBdy2Grnd)
  gradientDist/1 -> Gradient Based Derivative/2(gradDist)
  flowVelGradGrnd/1 -> Gradient Based Derivative/1(flowVelGradGrnd)
  [velVecBdy] -> Minus1/2
  velVecBdy/1 -> [velVecBdy]
  Mux/1 -> [nuRel]
  Minus1/1 -> Mux/1
  Matrix Multiply4/1 -> Mux2/1
  RGrnd2Bdy/1 -> Matrix Multiply4/1
  Mux2/1 -> [nuDotFlow]  "nuDotFlowEst"
  Constant3/1 -> Mux2/2
  Selector1/1 -> MAddedBdy/1
  Selector/1 -> FAddedBdy/1
  Add/1 -> Selector1/1, Selector/1
  [nuDotFlowTau] -> Add/1
  [relVelTau] -> Add/2
  Matrix Multiply1/1 -> [nuDotFlowTau]
  [nuDotFlow] -> Matrix Multiply1/2
  Constant2/1 -> Matrix Multiply1/1
  Matrix Multiply/1 -> [relVelTau]
  [nuRel] -> Matrix Multiply/2
  Subsystem/1(Ca) -> Matrix Multiply/1
  [nuRel] -> Subsystem/2(nuRel)
  Constant/1 -> Subsystem/1(Ma)
  "flowVelBdy "/1 -> Reshape/1
  angVelBdy/1 -> Mux/2

== system JoshTestingOCTModel/plant/vehicle/vehicleLETest/Subsystem ==
  FluidCentPosMat : Inport
  gradientDist : Inport  Port=2
  Add10 : Sum
  Constant1 : Constant  Value=ones(1,6)  VectorParams1D=off
  Constant2 : Constant  Value=eye(3)
  Gain1 : Gain  Gain=-1
  Matrix Multiply : Product  Multiplication=Matrix(*)
  Multiply2 : Product
  Selector2 : Selector  NumberOfDimensions=2  InputPortWidth=3  IndexOptions=Select all,Index vector (dialog)  Indices=[1 3],5  OutputSizes=1,1
  Vector Concatenate : Concatenate  Mode=Multidimensional array  ConcatenateDimension=2
  GradientFlowPos : Outport
  wires:
  gradientDist/1 -> Multiply2/1
  Add10/1 -> GradientFlowPos/1
  Constant2/1 -> Multiply2/2
  Gain1/1 -> Vector Concatenate/2
  Matrix Multiply/1 -> Add10/1
  Constant1/1 -> Matrix Multiply/2
  Multiply2/1 -> Vector Concatenate/1, Gain1/1
  Selector2/1 -> Matrix Multiply/1
  Vector Concatenate/1 -> Add10/2
  FluidCentPosMat/1 -> Selector2/1

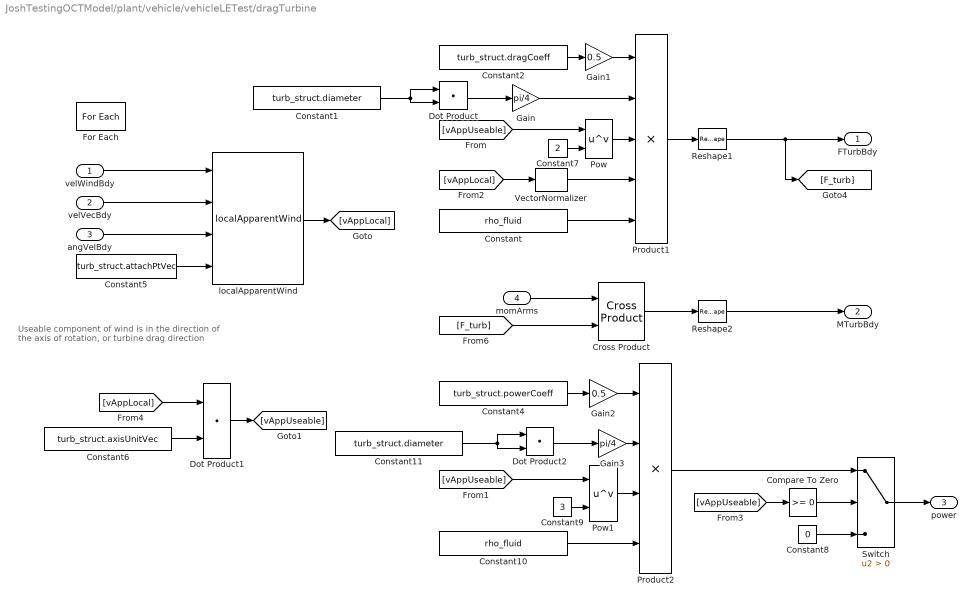
== system JoshTestingOCTModel/plant/vehicle/vehicleLETest/dragTurbine ==
  note: Useable component of wind is in the direction of
      | the axis of rotation, or turbine drag direction
  velWindBdy : Inport
  velVecBdy : Inport  Port=2
  angVelBdy : Inport  Port=3
  momArms : Inport  Port=4
  Compare To Zero : simulink/Logic and Bit Operations/Compare To Zero  relop=>=  OutDataTypeStr=boolean
  Constant : Constant  Value=rho_fluid
  Constant1 : Constant  Value=turb_struct.diameter  VectorParams1D=off
  Constant10 : Constant  Value=rho_fluid
  Constant11 : Constant  Value=turb_struct.diameter  VectorParams1D=off
  Constant2 : Constant  Value=turb_struct.dragCoeff  VectorParams1D=off
  Constant4 : Constant  Value=turb_struct.powerCoeff  VectorParams1D=off
  Constant5 : Constant  Value=turb_struct.attachPtVec
  Constant6 : Constant  Value=turb_struct.axisUnitVec
  Constant7 : Constant  Value=2
  Constant8 : Constant  Value=0
  Constant9 : Constant  Value=3
  Cross Product : vrlib/Utilities/Cross Product
      settings: SourceProductBaseCode=VR
  Dot Product : DotProduct  InputSameDT=on  OutDataTypeStr=Inherit: Inherit via internal rule
  Dot Product1 : DotProduct  InputSameDT=on  OutDataTypeStr=Inherit: Inherit via internal rule
  Dot Product2 : DotProduct  InputSameDT=on  OutDataTypeStr=Inherit: Inherit via internal rule
  For Each : ForEach  DisableCoverage=on  IterateSubsysMaskParameter=off,on,off  SubsysMaskParameterIterationDimension=1,2,1  IndexMode=One-based
  Gain : Gain  Gain=pi/4
  Gain1 : Gain  Gain=0.5
  Gain2 : Gain  Gain=0.5
  Gain3 : Gain  Gain=pi/4
  Pow : Math  Operator=pow  RndMeth=Zero  SaturateOnIntegerOverflow=on
  Pow1 : Math  Operator=pow  RndMeth=Zero  SaturateOnIntegerOverflow=on
  Product1 : Product  Inputs=5
  Product2 : Product  Inputs=4
  Reshape1 : Reshape  OutputDimensionality=Column vector (2-D)
  Reshape2 : Reshape  OutputDimensionality=Column vector (2-D)
  Switch : Switch  Criteria=u2 > Threshold
  "VectorNormalizer " : vectorNormalizer_ul/VectorNormalizer   SystemSampleTime=-1
  localApparentWind : localApparentWind_ul/localApparentWind  SystemSampleTime=-1
  FTurbBdy : Outport  PortDimensions=[3,1]  ConcatenationDimension=2
  MTurbBdy : Outport  Port=2  PortDimensions=[3,1]  ConcatenationDimension=2
  power : Outport  Port=3  PortDimensions=[1,1]  ConcatenationDimension=2
  wires:
  Gain3/1 -> Product2/2
  Constant11/1 -> Dot Product2/1, Dot Product2/2
  Dot Product2/1 -> Gain3/1
  Gain/1 -> Product1/2
  Dot Product/1 -> Gain/1
  [vAppUseable] -> Pow1/1
  [vAppLocal] -> Dot Product1/1
  Constant8/1 -> Switch/3
  [vAppUseable] -> Compare To Zero/1
  Compare To Zero/1 -> Switch/2
  Switch/1 -> power/1
  [vAppLocal] -> "VectorNormalizer "/1
  Constant7/1 -> Pow/2
  Pow/1 -> Product1/3
  Pow1/1 -> Product2/3
  Constant4/1 -> Gain2/1
  Gain2/1 -> Product2/1
  Constant10/1 -> Product2/4
  Constant/1 -> Product1/5
  Gain1/1 -> Product1/1
  Dot Product1/1 -> [vAppUseable]
  Constant9/1 -> Pow1/2
  Constant1/1 -> Dot Product/2, Dot Product/1
  "VectorNormalizer "/1 -> Product1/4
  [vAppUseable] -> Pow/1
  Constant6/1 -> Dot Product1/2
  Constant5/1 -> localApparentWind/4
  localApparentWind/1 -> [vAppLocal]
  velWindBdy/1 -> localApparentWind/1
  angVelBdy/1 -> localApparentWind/3
  velVecBdy/1 -> localApparentWind/2
  Reshape2/1 -> MTurbBdy/1
  Reshape1/1 -> [F_turb], FTurbBdy/1
  [F_turb] -> Cross Product/2
  momArms/1 -> Cross Product/1
  Constant2/1 -> Gain1/1
  Product2/1 -> Switch/1
  Product1/1 -> Reshape1/1
  Cross Product/1 -> Reshape2/1

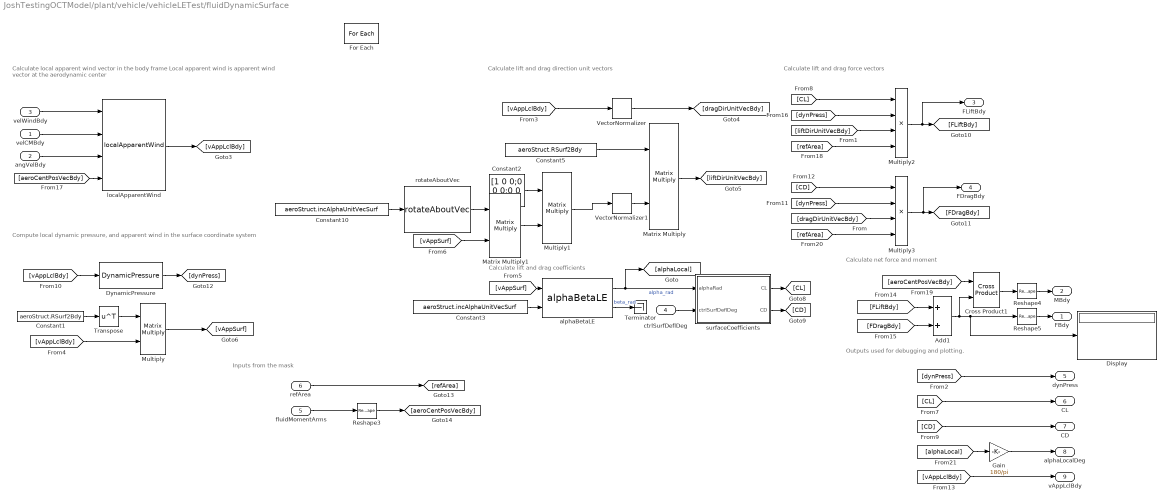
== system JoshTestingOCTModel/plant/vehicle/vehicleLETest/fluidDynamicSurface ==
  note: Calculate local apparent wind vector in the body frame
      | Local apparent wind is apparent wind vector at the aerodynamic center
  note: Calculate lift and drag direction unit vectors
  note: Inputs from the mask
  note: Compute local dynamic pressure,
      | and apparent wind in the surface coordinate system
  note: Calculate lift and drag coefficients
  note: Calculate lift and drag force vectors
  note: Calculate net force and moment
  note: Outputs used for debugging and plotting.
  velCMBdy : Inport
  angVelBdy : Inport  Port=2
  velWindBdy : Inport  Port=3  Partition=on  PartitionDimension=2  PartitionWidth=1  PartitionOffset=0
  ctrlSurfDeflDeg : Inport  Port=4  Partition=on  PartitionDimension=1  PartitionWidth=1  PartitionOffset=0
  fluidMomentArms : Inport  Port=5  Partition=on  PartitionDimension=2  PartitionWidth=1  PartitionOffset=0
  refArea : Inport  Port=6
  Add1 : Sum
  Constant1 : Constant  Value=aeroStruct.RSurf2Bdy
  Constant10 : Constant  Value=aeroStruct.incAlphaUnitVecSurf
  Constant2 : Constant  Value=[1 0 0;0 0 0;0 0 1]
  Constant3 : Constant  Value=aeroStruct.incAlphaUnitVecSurf
  Constant5 : Constant  Value=aeroStruct.RSurf2Bdy
  Cross Product1 : vrlib/Utilities/Cross Product
      settings: SourceProductBaseCode=VR
  Display : Display
  DynamicPressure : dynamicPressure_ul/DynamicPressure  rho=fluidDensity
  For Each : ForEach  DisableCoverage=on  IterateSubsysMaskParameter=on,off  SubsysMaskParameterIterationDimension=2,1  IndexMode=One-based
  Gain : Gain  Gain=180/pi
  Matrix Multiply : Product  Multiplication=Matrix(*)
  Matrix Multiply1 : Product  Multiplication=Matrix(*)
  Multiply : Product  Multiplication=Matrix(*)
  Multiply1 : Product  Multiplication=Matrix(*)
  Multiply2 : Product  Inputs=4
  Multiply3 : Product  Inputs=4
  Reshape3 : Reshape  OutputDimensionality=Column vector (2-D)
  Reshape4 : Reshape  OutputDimensionality=Column vector (2-D)
  Reshape5 : Reshape  OutputDimensionality=Column vector (2-D)
  Terminator : Terminator
  Transpose : Math  Operator=transpose  SaturateOnIntegerOverflow=on
  "VectorNormalizer " : vectorNormalizer_ul/VectorNormalizer   SystemSampleTime=-1
  VectorNormalizer1 : vectorNormalizer_ul/VectorNormalizer   SystemSampleTime=-1
  alphaBetaLE : alphaBetaLE_ul/alphaBetaLE  SystemSampleTime=-1
  localApparentWind : localApparentWind_ul/localApparentWind  SystemSampleTime=-1
  rotateAboutVec : rotateAboutVec/rotateAboutVec  ang=90
  surfaceCoefficients : Subsystem  AncestorBlock=surfaceCoefficients_ul/surfaceCoefficients
  FBdy : Outport  ConcatenationDimension=2
  MBdy : Outport  Port=2  PortDimensions=[3 1]  ConcatenationDimension=2
  FLiftBdy : Outport  Port=3  ConcatenationDimension=2
  FDragBdy : Outport  Port=4  ConcatenationDimension=2
  dynPress : Outport  Port=5  ConcatenationDimension=2
  CL : Outport  Port=6  ConcatenationDimension=2
  CD : Outport  Port=7  ConcatenationDimension=2
  alphaLocalDeg : Outport  Port=8  ConcatenationDimension=2
  vAppLclBdy : Outport  Port=9  ConcatenationDimension=2
  wires:
  [alphaLocal] -> Gain/1
  [vAppLclBdy] -> vAppLclBdy/1
  Gain/1 -> alphaLocalDeg/1
  [CL] -> CL/1
  [CD] -> CD/1
  [dynPress] -> dynPress/1
  localApparentWind/1 -> [vAppLclBdy]
  [aeroCentPosVecBdy] -> localApparentWind/4
  angVelBdy/1 -> localApparentWind/3
  velCMBdy/1 -> localApparentWind/2
  alphaBetaLE/1 -> [alphaLocal], surfaceCoefficients/1(alphaRad)  "alpha_rad"
  ctrlSurfDeflDeg/1 -> surfaceCoefficients/2(ctrlSurfDeflDeg)
  Reshape5/1 -> FBdy/1
  Reshape4/1 -> MBdy/1
  Reshape3/1 -> [aeroCentPosVecBdy]
  refArea/1 -> [refArea]
  [aeroCentPosVecBdy] -> Cross Product1/1
  [refArea] -> Multiply3/4
  [refArea] -> Multiply2/4
  fluidMomentArms/1 -> Reshape3/1
  Cross Product1/1 -> Reshape4/1
  [dynPress] -> Multiply2/2
  VectorNormalizer1/1 -> Matrix Multiply/2
  Constant5/1 -> Matrix Multiply/1
  Matrix Multiply/1 -> [liftDirUnitVecBdy]
  [FLiftBdy] -> Add1/1
  [FDragBdy] -> Add1/2
  Add1/1 -> Cross Product1/2, Display/1, Reshape5/1
  [CD] -> Multiply3/1
  [dynPress] -> Multiply3/2
  [dragDirUnitVecBdy] -> Multiply3/3
  Multiply3/1 -> [FDragBdy], FDragBdy/1
  Multiply2/1 -> [FLiftBdy], FLiftBdy/1
  [vAppLclBdy] -> DynamicPressure/1
  [liftDirUnitVecBdy] -> Multiply2/3
  DynamicPressure/1 -> [dynPress]
  [CL] -> Multiply2/1
  surfaceCoefficients/2(CD) -> [CD]
  surfaceCoefficients/1(CL) -> [CL]
  alphaBetaLE/2 -> Terminator/1  "beta_rad"
  [vAppSurf] -> alphaBetaLE/1
  Multiply/1 -> [vAppSurf]
  [vAppLclBdy] -> Multiply/2
  Constant1/1 -> Transpose/1
  "VectorNormalizer "/1 -> [dragDirUnitVecBdy]
  [vAppLclBdy] -> "VectorNormalizer "/1
  velWindBdy/1 -> localApparentWind/1
  Transpose/1 -> Multiply/1
  [vAppSurf] -> Matrix Multiply1/2
  rotateAboutVec/1 -> Matrix Multiply1/1
  Constant2/1 -> Multiply1/1
  Matrix Multiply1/1 -> Multiply1/2
  Multiply1/1 -> VectorNormalizer1/1
  Constant10/1 -> rotateAboutVec/1
  Constant3/1 -> alphaBetaLE/2

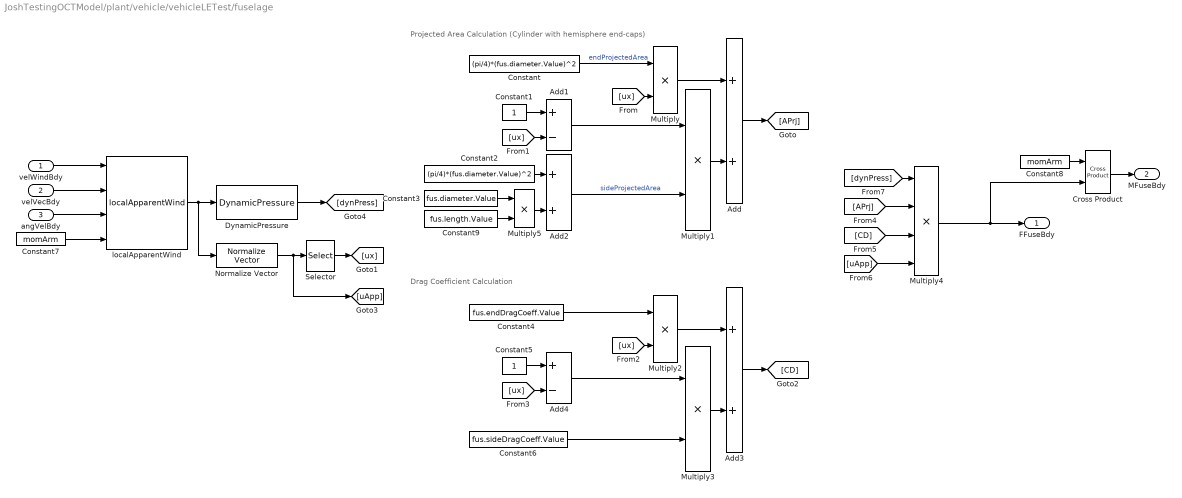
== system JoshTestingOCTModel/plant/vehicle/vehicleLETest/fuselage ==
  note: Projected Area Calculation (Cylinder with hemisphere end-caps)
  note: Drag Coefficient Calculation
  velWindBdy : Inport
  velVecBdy : Inport  Port=2
  angVelBdy : Inport  Port=3
  Add : Sum
  Add1 : Sum  Inputs=+-
  Add2 : Sum
  Add3 : Sum
  Add4 : Sum  Inputs=+-
  Constant : Constant  Value=(pi/4)*(fus.diameter.Value)^2
  Constant1 : Constant
  Constant2 : Constant  Value=(pi/4)*(fus.diameter.Value)^2
  Constant3 : Constant  Value=fus.diameter.Value
  Constant4 : Constant  Value=fus.endDragCoeff.Value
  Constant5 : Constant
  Constant6 : Constant  Value=fus.sideDragCoeff.Value
  Constant7 : Constant  Value=momArm
  Constant8 : Constant  Value=momArm
  Constant9 : Constant  Value=fus.length.Value
  Cross Product : vrlib/Utilities/Cross Product
      settings: SourceProductBaseCode=VR
  DynamicPressure : dynamicPressure_ul/DynamicPressure  rho=fusRhoDa
  Multiply{,1..3,5} (5 alike) : Product
  Multiply4 : Product  Inputs=4
  Normalize Vector : vrlib/Utilities/Normalize Vector  maxzero=0
      settings: SourceProductName=Simulink 3D Animation  SourceProductBaseCode=VR
  Selector : Selector  InputPortWidth=3  IndexOptions=Index vector (dialog)  Indices=1  OutputSizes=1
  localApparentWind : localApparentWind_ul/localApparentWind  SystemSampleTime=-1
  FFuseBdy : Outport
  MFuseBdy : Outport  Port=2
  wires:
  Constant9/1 -> Multiply5/2
  Constant3/1 -> Multiply5/1
  Multiply5/1 -> Add2/2
  Cross Product/1 -> MFuseBdy/1
  Constant8/1 -> Cross Product/1
  DynamicPressure/1 -> [dynPress]
  velWindBdy/1 -> localApparentWind/1
  Constant7/1 -> localApparentWind/4
  velVecBdy/1 -> localApparentWind/2
  localApparentWind/1 -> DynamicPressure/1, Normalize Vector/1
  angVelBdy/1 -> localApparentWind/3
  [uApp] -> Multiply4/4
  [CD] -> Multiply4/3
  [APrj] -> Multiply4/2
  [dynPress] -> Multiply4/1
  Multiply4/1 -> FFuseBdy/1, Cross Product/2
  Add3/1 -> [CD]
  Constant4/1 -> Multiply2/1
  Constant6/1 -> Multiply3/2
  Multiply3/1 -> Add3/2
  Multiply2/1 -> Add3/1
  [ux] -> Multiply2/2
  Add4/1 -> Multiply3/1
  Constant5/1 -> Add4/1
  [ux] -> Add4/2
  Constant2/1 -> Add2/1
  Add2/1 -> Multiply1/2  "sideProjectedArea"
  [ux] -> Add1/2
  Constant1/1 -> Add1/1
  Add1/1 -> Multiply1/1
  [ux] -> Multiply/2
  Constant/1 -> Multiply/1  "endProjectedArea"
  Multiply/1 -> Add/1
  Multiply1/1 -> Add/2
  Selector/1 -> [ux]
  Add/1 -> [APrj]
  Normalize Vector/1 -> Selector/1, [uApp]

== system JoshTestingOCTModel/plant/vehicle/vehicleLETest/sixDoFDynamics ==
  note: 1) Add Subsystem or Model blocks as valid variant choices.
      | 2) You cannot connect blocks at this level. At simulation, connectivity is automatically
      | determined, based on the active variant and port name matching.
  FNetBdy : Inport
  MNetBdy : Inport  Port=2
  SixDoFDynamicsQuat : SixDoFDynamicsQuat_ul/SixDoFDynamicsQuat  VariantControl=VSS_sixDoFDynamics_sixDoFDynamicsQuat  M=vcl.mass.Value  J=vcl.inertia.Value  initPos=vcl.initPosVecGnd.Value  initVel=vcl.initVelVecBdy.Value  initEulAngs=vcl.initEulAng.Value  initAngVel=vcl.initAngVelVec.Value
  sixDoFDynamicsCoupled : Subsystem  AncestorBlock=sixDoFDynamicsCoupled/sixDoFDynamicsCoupled  VariantControl=VSS_sixDoFDynamics_sixDoFDynamicsCoupled  mask{MMat=vcl.M6x6_B.Value, MaMat=vcl.Ma6x6_B.Value, rCM_B=vcl.rCM_B.Value, initPos=vcl.initPosVecGnd.Value, initVel=vcl.initVelVecBdy.Value, initEulAngs=vcl.initEulAng.Value, initAngVel=vcl.initAngVelVec.Value}
      mask prompts: MMat "6x6 Mass Matrix"; MaMat "6x6 Added Mass Matrix"; rCM_B "Center of mass position vec in body frame"; initPos "Initial position"; initVel "Initial velocity"; initEulAngs "Initial Euler Angles"; initAngVel "Initial Angular Velocity Vec"
      mask init:
      | MTot = MMat + MaMat;
      | MTotInv = inv(MTot);
      | 
      | m = MMat(1,1);
      | J = MMat(4:6,4:6);%About Body Frame
      mask DialogControl Container6 Prompt: Mass Matrices
      mask DialogControl Container4 Prompt: Point Locations
      mask DialogControl Container3 Prompt: Initial Conditions
  sixDoFDynamicsEuler : sixDoFDynamicsEuler_ul/sixDoFDynamicsEuler  VariantControl=VSS_sixDoFDynamics_sixDoFDynamicsEuler  M=vcl.mass.Value  J=vcl.inertia.Value  initPos=vcl.initPosVecGnd.Value  initVel=vcl.initVelVecBdy.Value  initEulAngs=vcl.initEulAng.Value  initAngVel=vcl.initAngVelVec.Value
  posVecGnd : Outport
  velVecGnd : Outport  Port=2
  eulerAngles : Outport  Port=3
  angularVel : Outport  Port=4
  Rinert2Bdy : Outport  Port=5
  RBdy2Inert : Outport  Port=6

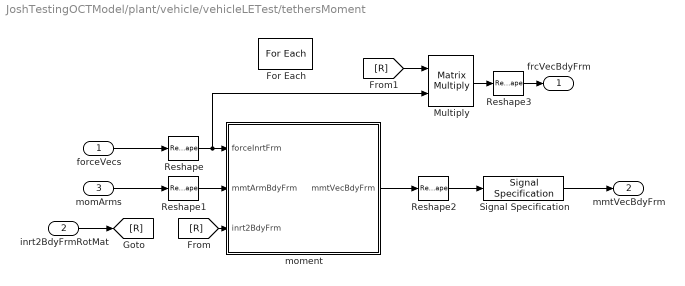
== system JoshTestingOCTModel/plant/vehicle/vehicleLETest/tethersMoment ==
  forceVecs : Inport  Partition=on  PartitionDimension=3  PartitionWidth=1  PartitionOffset=0
  inrt2BdyFrmRotMat : Inport  Port=2
  momArms : Inport  Port=3  Partition=on  PartitionDimension=2  PartitionWidth=1  PartitionOffset=0
  For Each : ForEach  DisableCoverage=on  IterateSubsysMaskParameter=on  SubsysMaskParameterIterationDimension=2  IndexMode=One-based
  Multiply : Product  Multiplication=Matrix(*)
  Reshape{,1..3} (4 alike) : Reshape  OutputDimensionality=Column vector (2-D)
  Signal Specification : SignalSpecification  Dimensions=[3 1]
  moment : Subsystem
  frcVecBdyFrm : Outport  ConcatenationDimension=2
  mmtVecBdyFrm : Outport  Port=2  ConcatenationDimension=2
  wires:
  Signal Specification/1 -> mmtVecBdyFrm/1
  Reshape3/1 -> frcVecBdyFrm/1
  Reshape2/1 -> Signal Specification/1
  Reshape1/1 -> moment/2(mmtArmBdyFrm)
  [R] -> Multiply/1
  Multiply/1 -> Reshape3/1
  [R] -> moment/3(inrt2BdyFrm)
  forceVecs/1 -> Reshape/1
  momArms/1 -> Reshape1/1
  inrt2BdyFrmRotMat/1 -> [R]
  moment/1(mmtVecBdyFrm) -> Reshape2/1
  Reshape/1 -> moment/1(forceInrtFrm), Multiply/2

== system JoshTestingOCTModel/plant/vehicle/vehicleLETest/thrAttachPtKinematics1 ==
  note: same as moment arms
      | for tether moments
  position : Inport
  velocity : Inport  Port=2
  angVel : Inport  Port=3
  bdy2GndRotMat : Inport  Port=4
  Add : Sum
  Add1 : Sum
  Bus Creator : BusCreator  Inputs=2  OutDataTypeStr=Bus: thrAttachPtKinematicsBus  NonVirtualBus=on
  Constant : Constant  Value=[0 0 0]
  Constant1 : Constant  Commented=on  Value=atchPts.rThrAttch_LE
  Constant2 : Constant  Value=zeros(3,1)
  For Each : ForEach  DisableCoverage=on  IterateSubsysMaskParameter=on  SubsysMaskParameterIterationDimension=2  IndexMode=One-based
  Multiply1 : Product  Multiplication=Matrix(*)
  Multiply3 : Product  Multiplication=Matrix(*)
  Reshape : Reshape  OutputDimensionality=Column vector (2-D)
  firstOrdTrnsThm : firstOrdTrnsThm_ul/firstOrdTrnsThm  SystemSampleTime=-1
  thrAttchPtBusArry : Outport  ConcatenationDimension=1
  wires:
  Add1/1 -> Bus Creator/1  "posVec"
  Add/1 -> Bus Creator/2  "velVec"
  bdy2GndRotMat/1 -> Multiply3/1, Multiply1/1
  Constant/1 -> firstOrdTrnsThm/2
  firstOrdTrnsThm/1 -> Multiply1/2
  angVel/1 -> firstOrdTrnsThm/3
  Constant2/1 -> Reshape/1
  Bus Creator/1 -> thrAttchPtBusArry/1
  position/1 -> Add1/1
  velocity/1 -> Add/1
  Multiply1/1 -> Add/2  "velVec"
  Multiply3/1 -> Add1/2  "posVec"
  Reshape/1 -> Multiply3/2, firstOrdTrnsThm/1

== system JoshTestingOCTModel/plant/vehicle/vehicleLETest/Non-Body-Inertial Added Mass/FilteredDiscreteDerivative ==
  flowVecGrnd : Inport
  Clock : Clock
  Divide : Product  Inputs=*/
  Memory : Memory
  Memory1 : Memory  InitialCondition=-.01
  Minus : Sum  Inputs=+-
  Minus2 : Sum  Inputs=+-
  firstOrderFilter : firstOrderFilter_ul/firstOrderFilter  tau=.01  ic=zeros(3,1)
  nuDotFlowEstG : Outport
  wires:
  firstOrderFilter/1 -> nuDotFlowEstG/1  "nuDotFlowEstG"
  Memory/1 -> Minus/2
  Minus/1 -> Divide/1
  Memory1/1 -> Minus2/2
  Clock/1 -> Memory1/1, Minus2/1
  Minus2/1 -> Divide/2  "samp"
  flowVecGrnd/1 -> Memory/1, Minus/1
  Divide/1 -> firstOrderFilter/1

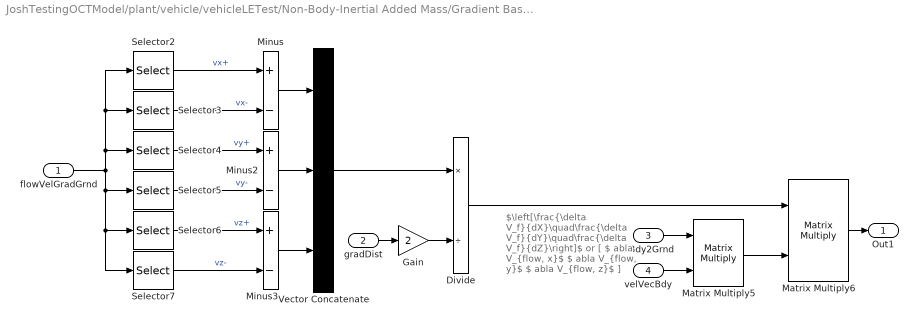
== system JoshTestingOCTModel/plant/vehicle/vehicleLETest/Non-Body-Inertial Added Mass/Gradient Based Derivative ==
  note: $\left[\frac{\delta V_f}{dX}\quad\frac{\delta V_f}{dY}\quad\frac{\delta V_f}{dZ}\right]$
      | or
      | [ $\nabla V_{flow, x}$
      | $\nabla V_{flow, y}$
      | $\nabla V_{flow, z}$ ]
  flowVelGradGrnd : Inport
  gradDist : Inport  Port=2
  RBdy2Grnd : Inport  Port=3
  velVecBdy : Inport  Port=4
  Divide : Product  Inputs=*/
  Gain : Gain  Gain=2
  Matrix Multiply5 : Product  Multiplication=Matrix(*)
  Matrix Multiply6 : Product  Multiplication=Matrix(*)
  Minus : Sum  Inputs=+-
  Minus2 : Sum  Inputs=+-
  Minus3 : Sum  Inputs=+-
  Selector2 : Selector  NumberOfDimensions=2  InputPortWidth=3  IndexOptions=Select all,Index vector (dialog)  Indices=[1 3],1  OutputSizes=1,1
  Selector3 : Selector  NumberOfDimensions=2  InputPortWidth=3  IndexOptions=Select all,Index vector (dialog)  Indices=[1 3],4  OutputSizes=1,1
  Selector4 : Selector  NumberOfDimensions=2  InputPortWidth=3  IndexOptions=Select all,Index vector (dialog)  Indices=[1 3],2  OutputSizes=1,1
  Selector5 : Selector  NumberOfDimensions=2  InputPortWidth=3  IndexOptions=Select all,Index vector (dialog)  Indices=[1 3],5  OutputSizes=1,1
  Selector6 : Selector  NumberOfDimensions=2  InputPortWidth=3  IndexOptions=Select all,Index vector (dialog)  Indices=[1 3],3  OutputSizes=1,1
  Selector7 : Selector  NumberOfDimensions=2  InputPortWidth=3  IndexOptions=Select all,Index vector (dialog)  Indices=[1 3],1  OutputSizes=1,1
  Vector Concatenate : Concatenate  NumInputs=3  Mode=Multidimensional array  ConcatenateDimension=2
  Out1 : Outport
  wires:
  Matrix Multiply6/1 -> Out1/1
  Divide/1 -> Matrix Multiply6/1
  Selector2/1 -> Minus/1  "vx+"
  Selector3/1 -> Minus/2  "vx-"
  RBdy2Grnd/1 -> Matrix Multiply5/1
  Gain/1 -> Divide/2
  Minus3/1 -> Vector Concatenate/3
  flowVelGradGrnd/1 -> Selector7/1, Selector6/1, Selector5/1, Selector2/1, Selector3/1, Selector4/1
  Selector5/1 -> Minus2/2  "vy-"
  gradDist/1 -> Gain/1
  Selector4/1 -> Minus2/1  "vy+"
  Selector6/1 -> Minus3/1  "vz+"
  Vector Concatenate/1 -> Divide/1
  Minus2/1 -> Vector Concatenate/2
  Selector7/1 -> Minus3/2  "vz-"
  Matrix Multiply5/1 -> Matrix Multiply6/2
  Minus/1 -> Vector Concatenate/1
  velVecBdy/1 -> Matrix Multiply5/2

== system JoshTestingOCTModel/plant/vehicle/vehicleLETest/Non-Body-Inertial Added Mass/Subsystem ==
  Ma : Inport
  nuRel : Inport  Port=2
  Constant2 : Constant  Value=zeros(3)
  Cross Product Mat : xProdMatrix_ul/Cross Product Mat  SystemSampleTime=-1
  Cross Product Mat1 : xProdMatrix_ul/Cross Product Mat  SystemSampleTime=-1
  Gain : Gain  Gain=-1
  Gain1 : Gain  Gain=-1
  Matrix Multiply : Product  Multiplication=Matrix(*)
  Selector : Selector  InputPortWidth=6  IndexOptions=Index vector (dialog)  Indices=[1 2 3]  OutputSizes=1
  Selector1 : Selector  InputPortWidth=6  IndexOptions=Index vector (dialog)  Indices=[4 5 6]  OutputSizes=1
  Vector Concatenate : Concatenate  Mode=Multidimensional array  ConcatenateDimension=2
  Vector Concatenate1 : Concatenate  Mode=Multidimensional array  ConcatenateDimension=2
  Vector Concatenate2 : Concatenate  Mode=Multidimensional array
  Ca : Outport
  wires:
  Vector Concatenate2/1 -> Ca/1
  nuRel/1 -> Matrix Multiply/2
  Constant2/1 -> Vector Concatenate/1
  Vector Concatenate/1 -> Vector Concatenate2/1
  Gain1/1 -> Vector Concatenate1/2
  Cross Product Mat/1 -> Gain/1
  Vector Concatenate1/1 -> Vector Concatenate2/2
  Cross Product Mat1/1 -> Gain1/1
  Selector1/1 -> Cross Product Mat1/1
  Matrix Multiply/1 -> Selector1/1, Selector/1
  Selector/1 -> Cross Product Mat/1
  Ma/1 -> Matrix Multiply/1
  Gain/1 -> Vector Concatenate/2, Vector Concatenate1/1
